simulink library "lib_BuildingThermalLiquid"  (R2026a)
settings: Solver=VariableStepAuto
libraries: ExternalWall_lib x47, WallSelector_lib x36, fl_lib x20, RoomWithRadiatorAndUFP x15
(part 5 of 5)

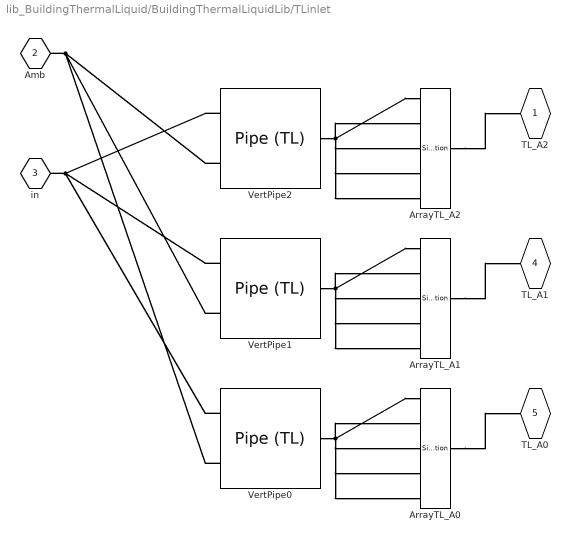
== system lib_BuildingThermalLiquid/BuildingThermalLiquidLib/TLinlet ==
  ArrayTL_A0 : SimscapeArrayConnection  Domain=foundation.thermal_liquid.thermal_liquid  ConcatenateDimension=1  NumScalarElements=5
  ArrayTL_A1 : SimscapeArrayConnection  Domain=foundation.thermal_liquid.thermal_liquid  ConcatenateDimension=1  NumScalarElements=5
  ArrayTL_A2 : SimscapeArrayConnection  Domain=foundation.thermal_liquid.thermal_liquid  ConcatenateDimension=1  NumScalarElements=5
  VertPipe0 : fl_lib/Thermal Liquid/Elements/Pipe (TL)  length=3.048 % Parameterized on : 11-Dec-2025 09:25:50 m  area=2.5e-05 % Parameterized on : 11-Dec-2025 09:25:50 m^2  Dh=0.005 % Parameterized on : 11-Dec-2025 09:25:50 m  length_add=0 % Parameterized on : 11-Dec-2025 09:25:50 m  roughness=15e-6 m  Re_lam=2000  Re_tur=4000  shape_factor=64  Nu_lam=3.66  dynamic_compressibility=true  inertia=false  p0=0.101325 MPa  T0=300 % Parameterized on : 11-Dec-2025 09:25:50 K  mdot0=0 kg/s  p_nominal=0.101325 MPa  T_nominal=293.15 K
  VertPipe1 : fl_lib/Thermal Liquid/Elements/Pipe (TL)  length=6.096 % Parameterized on : 11-Dec-2025 09:25:50 m  area=2.5e-05 % Parameterized on : 11-Dec-2025 09:25:50 m^2  Dh=0.005 % Parameterized on : 11-Dec-2025 09:25:50 m  length_add=0 % Parameterized on : 11-Dec-2025 09:25:50 m  roughness=15e-6 m  Re_lam=2000  Re_tur=4000  shape_factor=64  Nu_lam=3.66  dynamic_compressibility=true  inertia=false  p0=0.101325 MPa  T0=300 % Parameterized on : 11-Dec-2025 09:25:50 K  mdot0=0 kg/s  p_nominal=0.101325 MPa  T_nominal=293.15 K
  VertPipe2 : fl_lib/Thermal Liquid/Elements/Pipe (TL)  length=9.144 % Parameterized on : 11-Dec-2025 09:25:49 m  area=2.5e-05 % Parameterized on : 11-Dec-2025 09:25:50 m^2  Dh=0.005 % Parameterized on : 11-Dec-2025 09:25:50 m  length_add=0 % Parameterized on : 11-Dec-2025 09:25:50 m  roughness=15e-6 m  Re_lam=2000  Re_tur=4000  shape_factor=64  Nu_lam=3.66  dynamic_compressibility=true  inertia=false  p0=0.101325 MPa  T0=300 % Parameterized on : 11-Dec-2025 09:25:50 K  mdot0=0 kg/s  p_nominal=0.101325 MPa  T_nominal=293.15 K
  TL_A2 : PMIOPort  Side=Right
  Amb : PMIOPort  Port=2  Side=Left
  in : PMIOPort  Port=3  Side=Left
  TL_A1 : PMIOPort  Port=4  Side=Right
  TL_A0 : PMIOPort  Port=5  Side=Right
  connections:
  ArrayTL_A2/RConn1 -- TL_A2/RConn1
  ArrayTL_A2/LConn1 -- VertPipe2/RConn1 -- ArrayTL_A2/LConn2 -- ArrayTL_A2/LConn3 -- ArrayTL_A2/LConn4 -- ArrayTL_A2/LConn5
  VertPipe2/LConn1 -- VertPipe1/LConn1 -- in/RConn1 -- VertPipe0/LConn1
  VertPipe2/LConn2 -- VertPipe1/LConn2 -- Amb/RConn1 -- VertPipe0/LConn2
  ArrayTL_A1/RConn1 -- TL_A1/RConn1
  ArrayTL_A1/LConn1 -- VertPipe1/RConn1 -- ArrayTL_A1/LConn2 -- ArrayTL_A1/LConn3 -- ArrayTL_A1/LConn4 -- ArrayTL_A1/LConn5
  ArrayTL_A0/RConn1 -- TL_A0/RConn1
  ArrayTL_A0/LConn1 -- VertPipe0/RConn1 -- ArrayTL_A0/LConn2 -- ArrayTL_A0/LConn3 -- ArrayTL_A0/LConn4 -- ArrayTL_A0/LConn5

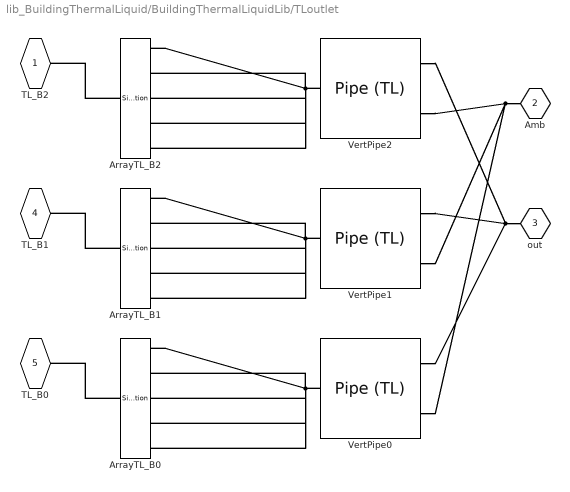
== system lib_BuildingThermalLiquid/BuildingThermalLiquidLib/TLoutlet ==
  ArrayTL_B0 : SimscapeArrayConnection  Domain=foundation.thermal_liquid.thermal_liquid  ConcatenateDimension=1  NumScalarElements=5
  ArrayTL_B1 : SimscapeArrayConnection  Domain=foundation.thermal_liquid.thermal_liquid  ConcatenateDimension=1  NumScalarElements=5
  ArrayTL_B2 : SimscapeArrayConnection  Domain=foundation.thermal_liquid.thermal_liquid  ConcatenateDimension=1  NumScalarElements=5
  VertPipe0 : fl_lib/Thermal Liquid/Elements/Pipe (TL)  length=3.048 % Parameterized on : 11-Dec-2025 09:25:50 m  area=2.5e-05 % Parameterized on : 11-Dec-2025 09:25:50 m^2  Dh=0.005 % Parameterized on : 11-Dec-2025 09:25:50 m  length_add=0 % Parameterized on : 11-Dec-2025 09:25:50 m  roughness=15e-6 m  Re_lam=2000  Re_tur=4000  shape_factor=64  Nu_lam=3.66  dynamic_compressibility=true  inertia=false  p0=0.101325 MPa  T0=300 % Parameterized on : 11-Dec-2025 09:25:50 K  mdot0=0 kg/s  p_nominal=0.101325 MPa  T_nominal=293.15 K
  VertPipe1 : fl_lib/Thermal Liquid/Elements/Pipe (TL)  length=6.096 % Parameterized on : 11-Dec-2025 09:25:50 m  area=2.5e-05 % Parameterized on : 11-Dec-2025 09:25:50 m^2  Dh=0.005 % Parameterized on : 11-Dec-2025 09:25:50 m  length_add=0 % Parameterized on : 11-Dec-2025 09:25:50 m  roughness=15e-6 m  Re_lam=2000  Re_tur=4000  shape_factor=64  Nu_lam=3.66  dynamic_compressibility=true  inertia=false  p0=0.101325 MPa  T0=300 % Parameterized on : 11-Dec-2025 09:25:50 K  mdot0=0 kg/s  p_nominal=0.101325 MPa  T_nominal=293.15 K
  VertPipe2 : fl_lib/Thermal Liquid/Elements/Pipe (TL)  length=9.144 % Parameterized on : 11-Dec-2025 09:25:50 m  area=2.5e-05 % Parameterized on : 11-Dec-2025 09:25:50 m^2  Dh=0.005 % Parameterized on : 11-Dec-2025 09:25:50 m  length_add=0 % Parameterized on : 11-Dec-2025 09:25:50 m  roughness=15e-6 m  Re_lam=2000  Re_tur=4000  shape_factor=64  Nu_lam=3.66  dynamic_compressibility=true  inertia=false  p0=0.101325 MPa  T0=300 % Parameterized on : 11-Dec-2025 09:25:50 K  mdot0=0 kg/s  p_nominal=0.101325 MPa  T_nominal=293.15 K
  TL_B2 : PMIOPort  Side=Left
  Amb : PMIOPort  Port=2  Side=Right
  out : PMIOPort  Port=3  Side=Right
  TL_B1 : PMIOPort  Port=4  Side=Left
  TL_B0 : PMIOPort  Port=5  Side=Left
  connections:
  ArrayTL_B2/RConn1 -- TL_B2/RConn1
  ArrayTL_B2/LConn1 -- VertPipe2/RConn1 -- ArrayTL_B2/LConn2 -- ArrayTL_B2/LConn3 -- ArrayTL_B2/LConn4 -- ArrayTL_B2/LConn5
  VertPipe2/LConn1 -- VertPipe1/LConn1 -- out/RConn1 -- VertPipe0/LConn1
  VertPipe2/LConn2 -- VertPipe1/LConn2 -- Amb/RConn1 -- VertPipe0/LConn2
  ArrayTL_B1/RConn1 -- TL_B1/RConn1
  ArrayTL_B1/LConn1 -- VertPipe1/RConn1 -- ArrayTL_B1/LConn2 -- ArrayTL_B1/LConn3 -- ArrayTL_B1/LConn4 -- ArrayTL_B1/LConn5
  ArrayTL_B0/RConn1 -- TL_B0/RConn1
  ArrayTL_B0/LConn1 -- VertPipe0/RConn1 -- ArrayTL_B0/LConn2 -- ArrayTL_B0/LConn3 -- ArrayTL_B0/LConn4 -- ArrayTL_B0/LConn5

== system lib_BuildingThermalLiquid/BuildingThermalLiquidLib/roomT ==
  concat1 : fl_lib/Physical Signals/Functions/PS Concatenate  catColumns=true
  concat2 : fl_lib/Physical Signals/Functions/PS Concatenate  catColumns=true
  1 : PMIOPort  Side=Left
  2 : PMIOPort  Port=2  Side=Left
  3 : PMIOPort  Port=3  Side=Left
  v : PMIOPort  Port=4  Side=Right
  connections:
  1/RConn1 -- concat1/LConn1
  2/RConn1 -- concat1/LConn2
  concat1/RConn1 -- concat2/LConn1
  3/RConn1 -- concat2/LConn2
  concat2/RConn1 -- v/RConn1

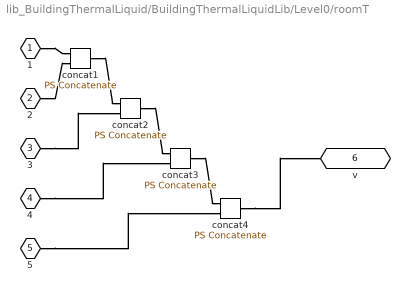
== system lib_BuildingThermalLiquid/BuildingThermalLiquidLib/Level0/roomT ==
  concat{1..4} (4 alike) : fl_lib/Physical Signals/Functions/PS Concatenate  catColumns=true
  1 : PMIOPort  Side=Left
  2 : PMIOPort  Port=2  Side=Left
  3 : PMIOPort  Port=3  Side=Left
  4 : PMIOPort  Port=4  Side=Left
  5 : PMIOPort  Port=5  Side=Left
  v : PMIOPort  Port=6  Side=Right
  connections:
  1/RConn1 -- concat1/LConn1
  2/RConn1 -- concat1/LConn2
  concat1/RConn1 -- concat2/LConn1
  3/RConn1 -- concat2/LConn2
  concat2/RConn1 -- concat3/LConn1
  4/RConn1 -- concat3/LConn2
  concat3/RConn1 -- concat4/LConn1
  5/RConn1 -- concat4/LConn2
  concat4/RConn1 -- v/RConn1

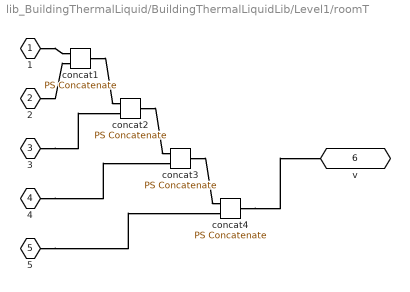
== system lib_BuildingThermalLiquid/BuildingThermalLiquidLib/Level1/roomT ==
  concat{1..4} (4 alike) : fl_lib/Physical Signals/Functions/PS Concatenate  catColumns=true
  1 : PMIOPort  Side=Left
  2 : PMIOPort  Port=2  Side=Left
  3 : PMIOPort  Port=3  Side=Left
  4 : PMIOPort  Port=4  Side=Left
  5 : PMIOPort  Port=5  Side=Left
  v : PMIOPort  Port=6  Side=Right
  connections:
  1/RConn1 -- concat1/LConn1
  2/RConn1 -- concat1/LConn2
  concat1/RConn1 -- concat2/LConn1
  3/RConn1 -- concat2/LConn2
  concat2/RConn1 -- concat3/LConn1
  4/RConn1 -- concat3/LConn2
  concat3/RConn1 -- concat4/LConn1
  5/RConn1 -- concat4/LConn2
  concat4/RConn1 -- v/RConn1

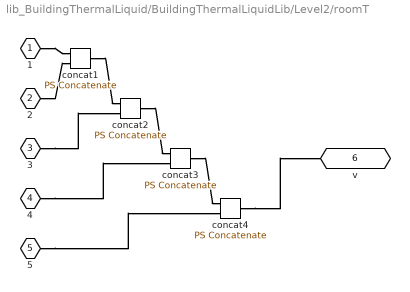
== system lib_BuildingThermalLiquid/BuildingThermalLiquidLib/Level2/roomT ==
  concat{1..4} (4 alike) : fl_lib/Physical Signals/Functions/PS Concatenate  catColumns=true
  1 : PMIOPort  Side=Left
  2 : PMIOPort  Port=2  Side=Left
  3 : PMIOPort  Port=3  Side=Left
  4 : PMIOPort  Port=4  Side=Left
  5 : PMIOPort  Port=5  Side=Left
  v : PMIOPort  Port=6  Side=Right
  connections:
  1/RConn1 -- concat1/LConn1
  2/RConn1 -- concat1/LConn2
  concat1/RConn1 -- concat2/LConn1
  3/RConn1 -- concat2/LConn2
  concat2/RConn1 -- concat3/LConn1
  4/RConn1 -- concat3/LConn2
  concat3/RConn1 -- concat4/LConn1
  5/RConn1 -- concat4/LConn2
  concat4/RConn1 -- v/RConn1
